simulink model "crash_predictor"  (Simulink 9.1)
settings: Solver=VariableStepAuto  StartTime=0.0  StopTime=10.0  RelTol=1e-3
values from neighbouring files (symbols this model uses):
  Estimator =     [data_set.mat]
libraries: F_Line_block x43, simulink x6
settings Model: Creator=dongw  LastModifiedBy=dongw
settings DataIOCC: SaveFormat=Dataset
settings OptimizationCC: LifeSpan=auto
settings DebuggingCC: UnderspecifiedInitializationDetection=Simplified  MergeDetectMultiDrivingBlocksExec=error  SFUnexpectedBacktrackingDiag=error  SFNoUnconditionalDefaultTransitionDiag=error  SFExecutionAtInitializationDiag=warning
settings HardwareCC: ProdBitPerPointer=64  ProdBitPerSizeT=64  ProdBitPerPtrDiffT=64  ProdLargestAtomicFloat=Float  ProdIntDivRoundTo=Zero  ProdEndianess=LittleEndian  ProdWordSize=64  ProdHWDeviceType=Intel->x86-64 (Windows64)
settings ModelReferenceCC: PropagateSignalLabelsOutOfModel=on
settings CodeAppCC: StateflowObjectComments=off
settings GRTTargetCC: TargetLangStandard=C99 (ISO)  CombineOutputUpdateFcns=on  GRTInterface=off
settings ConfigComp: CovMetricSettings=dwe  CovHtmlReporting=off  CovSaveCumulativeToWorkspaceVar=off  CovSaveSingleToWorkspaceVar=off  CovExternalEMLEnable=on

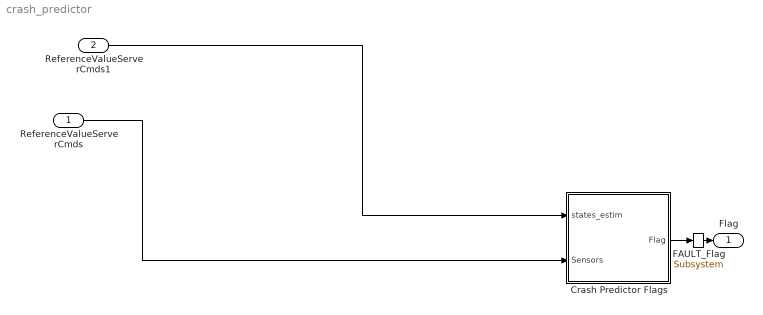
== system crash_predictor ==
  ReferenceValueServerCmds : Inport  OutDataTypeStr=Bus: CommandBus
  ReferenceValueServerCmds1 : Inport  Port=2  OutDataTypeStr=Bus: CommandBus
  Crash Predictor Flags : Subsystem
  Flag : Outport
  FAULT_Flag : F_Line_block/Subsystem
  wires:
  Crash Predictor Flags/1(Flag) -> FAULT_Flag/1
  FAULT_Flag/1 -> Flag/1
  ReferenceValueServerCmds/1 -> Crash Predictor Flags/2(Sensors)
  ReferenceValueServerCmds1/1 -> Crash Predictor Flags/1(states_estim)

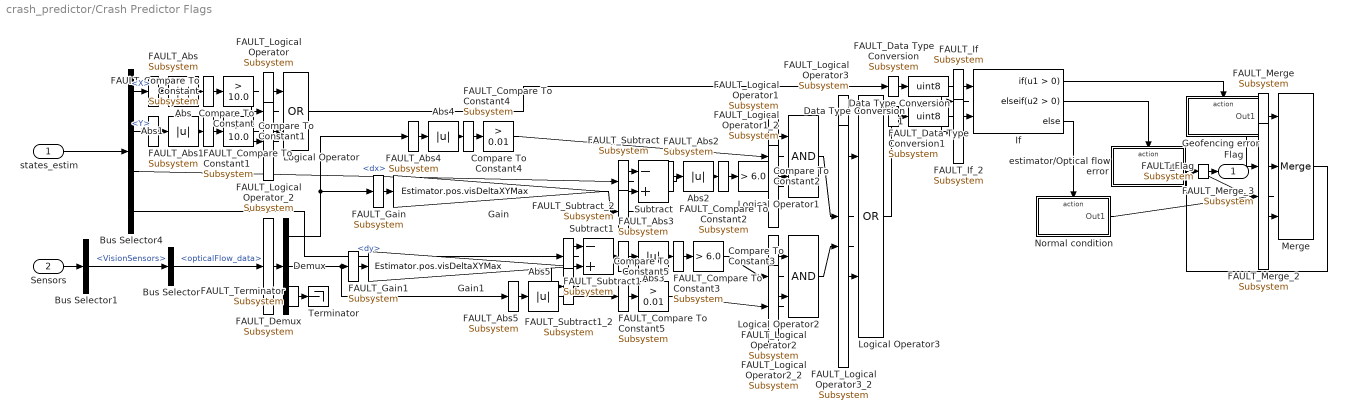
== system crash_predictor/Crash Predictor Flags ==
  states_estim : Inport
  Sensors : Inport  Port=2
  Abs{,1..5} (6 alike) : Abs
  FAULT_Abs{,1..5} (6 alike) : F_Line_block/Subsystem
  Bus Selector : BusSelector  OutputSignals=opticalFlow_data
  Bus Selector1 : BusSelector  OutputSignals=VisionSensors
  Bus Selector4 : BusSelector  OutputSignals=X,Y,dx,dy
  Compare To Constant : simulink/Logic and Bit Operations/Compare To Constant  relop=>  const=10.0  OutDataTypeStr=boolean
  FAULT_Compare To Constant{,1..5} (6 alike) : F_Line_block/Subsystem
  Compare To Constant1 : simulink/Logic and Bit Operations/Compare To Constant  relop=>  const=10.0  OutDataTypeStr=boolean
  Compare To Constant2 : simulink/Logic and Bit Operations/Compare To Constant  relop=>  const=6.0  OutDataTypeStr=boolean
  Compare To Constant3 : simulink/Logic and Bit Operations/Compare To Constant  relop=>  const=6.0  OutDataTypeStr=boolean
  Compare To Constant4 : simulink/Logic and Bit Operations/Compare To Constant  relop=>  const=0.01  OutDataTypeStr=boolean
  Compare To Constant5 : simulink/Logic and Bit Operations/Compare To Constant  relop=>  const=0.01  OutDataTypeStr=boolean
  Data Type Conversion : DataTypeConversion  OutDataTypeStr=uint8  RndMeth=Nearest
  FAULT_Data Type Conversion : F_Line_block/Subsystem
  Data Type Conversion1 : DataTypeConversion  OutDataTypeStr=uint8  RndMeth=Nearest
  FAULT_Data Type Conversion1 : F_Line_block/Subsystem
  Demux : Demux  Outputs=3
  FAULT_Demux : F_Line_block/Subsystem
  Gain : Gain  Gain=Estimator.pos.visDeltaXYMax
  FAULT_Gain : F_Line_block/Subsystem
  Gain1 : Gain  Gain=Estimator.pos.visDeltaXYMax
  FAULT_Gain1 : F_Line_block/Subsystem
  Geofencing error : Subsystem  TreatAsAtomicUnit=on
  If : If  NumInputs=2  ElseIfExpressions=u2 > 0
  FAULT_If : F_Line_block/Subsystem
  FAULT_If_2 : F_Line_block/Subsystem
  Logical Operator : Logic  Operator=OR  AllPortsSameDT=off
  FAULT_Logical Operator{,1..3} (4 alike) : F_Line_block/Subsystem
  FAULT_Logical Operator_2 : F_Line_block/Subsystem
  Logical Operator1 : Logic  AllPortsSameDT=off  OutDataTypeStr=boolean
  FAULT_Logical Operator1_2 : F_Line_block/Subsystem
  Logical Operator2 : Logic  AllPortsSameDT=off  OutDataTypeStr=boolean
  FAULT_Logical Operator2_2 : F_Line_block/Subsystem
  Logical Operator3 : Logic  Operator=OR  AllPortsSameDT=off
  FAULT_Logical Operator3_2 : F_Line_block/Subsystem
  Merge : Merge  Inputs=3  InitialOutput=0
  FAULT_Merge : F_Line_block/Subsystem
  FAULT_Merge_2 : F_Line_block/Subsystem
  FAULT_Merge_3 : F_Line_block/Subsystem
  Normal condition : Subsystem  TreatAsAtomicUnit=on
  Subtract : Sum  Inputs=-+
  FAULT_Subtract : F_Line_block/Subsystem
  FAULT_Subtract_2 : F_Line_block/Subsystem
  Subtract1 : Sum  Inputs=-+
  FAULT_Subtract1 : F_Line_block/Subsystem
  FAULT_Subtract1_2 : F_Line_block/Subsystem
  Terminator : Terminator
  FAULT_Terminator : F_Line_block/Subsystem
  estimator/Optical flow error : Subsystem  TreatAsAtomicUnit=on
  Flag : Outport
  FAULT_Flag : F_Line_block/Subsystem
  wires:
  Bus Selector4/1 -> FAULT_Abs/1  "<X>"
  FAULT_Abs/1 -> Abs/1
  states_estim/1 -> Bus Selector4/1
  Bus Selector4/2 -> FAULT_Abs1/1  "<Y>"
  FAULT_Abs1/1 -> Abs1/1
  Compare To Constant/1 -> FAULT_Logical Operator/1
  FAULT_Logical Operator/1 -> Logical Operator/1
  Compare To Constant1/1 -> FAULT_Logical Operator_2/1
  FAULT_Logical Operator_2/1 -> Logical Operator/2
  Abs/1 -> FAULT_Compare To Constant/1
  FAULT_Compare To Constant/1 -> Compare To Constant/1
  Abs1/1 -> FAULT_Compare To Constant1/1
  FAULT_Compare To Constant1/1 -> Compare To Constant1/1
  Logical Operator/1 -> FAULT_Data Type Conversion/1
  FAULT_Data Type Conversion/1 -> Data Type Conversion/1
  Bus Selector/1 -> FAULT_Demux/1  "<opticalFlow_data>"
  FAULT_Demux/1 -> Demux/1
  Demux/1 -> FAULT_Abs4/1, FAULT_Gain/1
  FAULT_Abs4/1 -> Abs4/1
  FAULT_Gain/1 -> Gain/1
  Demux/2 -> FAULT_Gain1/1, FAULT_Abs5/1
  FAULT_Gain1/1 -> Gain1/1
  FAULT_Abs5/1 -> Abs5/1
  Bus Selector4/3 -> FAULT_Subtract/1  "<dx>"
  FAULT_Subtract/1 -> Subtract/1
  Subtract/1 -> FAULT_Abs2/1
  FAULT_Abs2/1 -> Abs2/1
  Subtract1/1 -> FAULT_Abs3/1
  FAULT_Abs3/1 -> Abs3/1
  Abs2/1 -> FAULT_Compare To Constant2/1
  FAULT_Compare To Constant2/1 -> Compare To Constant2/1
  Abs3/1 -> FAULT_Compare To Constant3/1
  FAULT_Compare To Constant3/1 -> Compare To Constant3/1
  Compare To Constant5/1 -> FAULT_Logical Operator2_2/1
  FAULT_Logical Operator2_2/1 -> Logical Operator2/2
  Abs4/1 -> FAULT_Compare To Constant4/1
  FAULT_Compare To Constant4/1 -> Compare To Constant4/1
  Abs5/1 -> FAULT_Compare To Constant5/1
  FAULT_Compare To Constant5/1 -> Compare To Constant5/1
  Compare To Constant3/1 -> FAULT_Logical Operator2/1
  FAULT_Logical Operator2/1 -> Logical Operator2/1
  Logical Operator1/1 -> FAULT_Logical Operator3/1
  FAULT_Logical Operator3/1 -> Logical Operator3/1
  Logical Operator2/1 -> FAULT_Logical Operator3_2/1
  FAULT_Logical Operator3_2/1 -> Logical Operator3/2
  Logical Operator3/1 -> FAULT_Data Type Conversion1/1
  FAULT_Data Type Conversion1/1 -> Data Type Conversion1/1
  Demux/3 -> FAULT_Terminator/1
  FAULT_Terminator/1 -> Terminator/1
  Gain/1 -> FAULT_Subtract_2/1
  FAULT_Subtract_2/1 -> Subtract/2
  Bus Selector4/4 -> FAULT_Subtract1/1  "<dy>"
  FAULT_Subtract1/1 -> Subtract1/1
  Gain1/1 -> FAULT_Subtract1_2/1
  FAULT_Subtract1_2/1 -> Subtract1/2
  Compare To Constant4/1 -> FAULT_Logical Operator1/1
  FAULT_Logical Operator1/1 -> Logical Operator1/1
  Compare To Constant2/1 -> FAULT_Logical Operator1_2/1
  FAULT_Logical Operator1_2/1 -> Logical Operator1/2
  Sensors/1 -> Bus Selector1/1
  Bus Selector1/1 -> Bus Selector/1  "<VisionSensors>"
  Merge/1 -> FAULT_Flag/1
  FAULT_Flag/1 -> Flag/1
  If/1 -> Geofencing error/Action
  If/2 -> estimator/Optical flow error/Action
  If/3 -> Normal condition/Action
  Geofencing error/1(Out1) -> FAULT_Merge/1
  FAULT_Merge/1 -> Merge/1
  estimator/Optical flow error/1(Out1) -> FAULT_Merge_2/1
  FAULT_Merge_2/1 -> Merge/2
  Normal condition/1(Out1) -> FAULT_Merge_3/1
  FAULT_Merge_3/1 -> Merge/3
  Data Type Conversion/1 -> FAULT_If/1
  FAULT_If/1 -> If/1
  Data Type Conversion1/1 -> FAULT_If_2/1
  FAULT_If_2/1 -> If/2

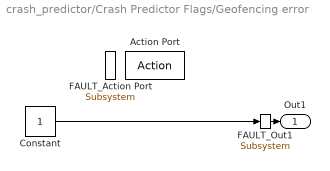
== system crash_predictor/Crash Predictor Flags/Geofencing error ==
  Action Port : ActionPort
  FAULT_Action Port : F_Line_block/Subsystem
  Constant : Constant  OutDataTypeStr=uint8
  Out1 : Outport
  FAULT_Out1 : F_Line_block/Subsystem
  wires:
  Constant/1 -> FAULT_Out1/1
  FAULT_Out1/1 -> Out1/1

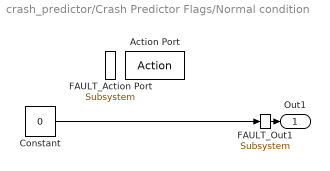
== system crash_predictor/Crash Predictor Flags/Normal condition ==
  Action Port : ActionPort
  FAULT_Action Port : F_Line_block/Subsystem
  Constant : Constant  Value=0  OutDataTypeStr=uint8
  Out1 : Outport
  FAULT_Out1 : F_Line_block/Subsystem
  wires:
  Constant/1 -> FAULT_Out1/1
  FAULT_Out1/1 -> Out1/1

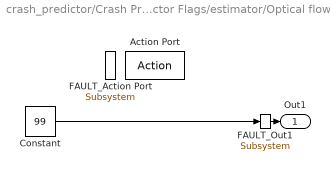
== system crash_predictor/Crash Predictor Flags/estimator/Optical flow error ==
  Action Port : ActionPort
  FAULT_Action Port : F_Line_block/Subsystem
  Constant : Constant  Value=99  OutDataTypeStr=uint8
  Out1 : Outport
  FAULT_Out1 : F_Line_block/Subsystem
  wires:
  Constant/1 -> FAULT_Out1/1
  FAULT_Out1/1 -> Out1/1
